simulink model "newsimul"  (R2023a)
settings: Solver=FixedStepAuto  StartTime=0.0  StopTime=51e-6 - 1/2e9  RelTol=1e-3
values from neighbouring files (symbols this model uses):
  yr_c = yr_c(t,:)    [matlab_channel.m]
undefined symbols (not defined in the file or in its folder): Add, Shift
libraries: hdlsllib x3, dsphdlfiltering2 x1, dsphdlmathfun2 x1
settings Model: Creator=Windows User  LastModifiedBy=Windows User
settings OptimizationCC: BlockReduction=off  ConditionallyExecuteInputs=off  DefaultParameterBehavior=Inlined
settings DebuggingCC: AlgebraicLoopMsg=error  SingleTaskRateTransMsg=error
settings HardwareCC: ProdBitPerPointer=32  ProdBitPerSizeT=32  ProdBitPerPtrDiffT=32  ProdLargestAtomicFloat=None  ProdIntDivRoundTo=Undefined  ProdEndianess=Unspecified  ProdWordSize=32  ProdHWDeviceType=ASIC/FPGA->ASIC/FPGA  TargetBitPerPointer=64  TargetBitPerSizeT=64  TargetBitPerPtrDiffT=64  TargetLongLongMode=on  TargetIntDivRoundTo=Zero  TargetEndianess=LittleEndian  TargetWordSize=64  TargetHWDeviceType=Custom Processor->MATLAB Host Computer  ProdEqTarget=off

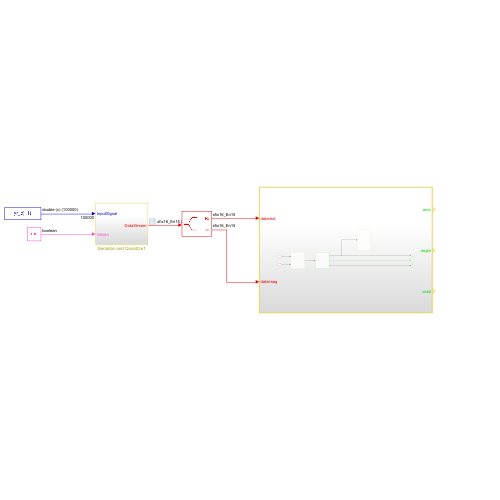
[thumbnail: Simulink's stored preview of the top-level diagram]
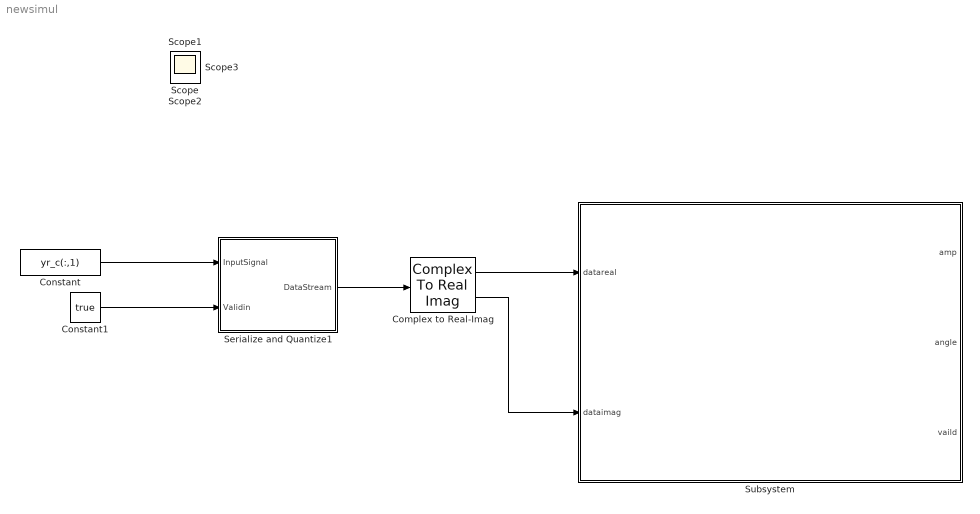
== system newsimul ==
  Complex to Real-Imag : ComplexToRealImag
  Constant : Constant  Value=yr_c(:,1)  SampleTime=50e-6
  Constant1 : Constant  Value=true  OutDataTypeStr=boolean
  Serialize and Quantize1 : Subsystem
  Subsystem : Subsystem  TreatAsAtomicUnit=on
  Scope{,1..3} (4 alike) : Scope
  wires:
  Constant1/1 -> Serialize and Quantize1/2(Validin)
  Serialize and Quantize1/1(DataStream) -> Complex to Real-Imag/1
  Complex to Real-Imag/1 -> Subsystem/1(datareal)
  Complex to Real-Imag/2 -> Subsystem/2(dataimag)
  Constant/1 -> Serialize and Quantize1/1(InputSignal)

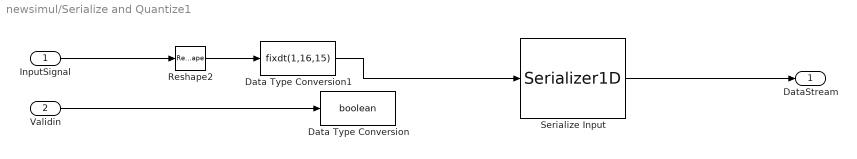
== system newsimul/Serialize and Quantize1 ==
  InputSignal : Inport
  Validin : Inport  Port=2
  Data Type Conversion : DataTypeConversion  OutDataTypeStr=boolean  SaturateOnIntegerOverflow=off  RndMeth=Floor
  Data Type Conversion1 : DataTypeConversion  OutDataTypeStr=fixdt(1,16,15)  RndMeth=Floor
  Reshape2 : Reshape  OutputDimensionality=Column vector (2-D)
  Serialize Input : hdlsllib/HDL Operations/Serializer1D  Ratio=100000  IdleCycles=0  validIn=off  startOut=off  validOut=off  inputDataDimensions=-1  inputSampleTime=-1  inputSignalType=auto
  DataStream : Outport
  wires:
  InputSignal/1 -> Reshape2/1
  Validin/1 -> Data Type Conversion/1
  Serialize Input/1 -> DataStream/1
  Reshape2/1 -> Data Type Conversion1/1
  Data Type Conversion1/1 -> Serialize Input/1

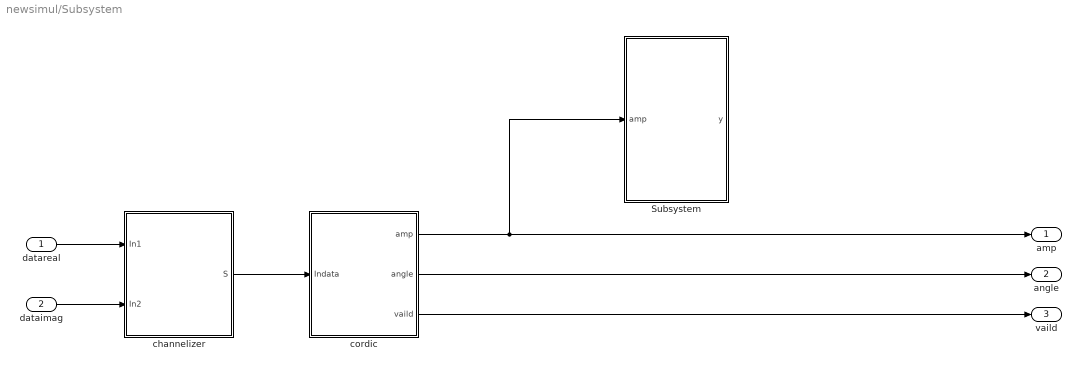
== system newsimul/Subsystem ==
  datareal : Inport
  dataimag : Inport  Port=2
  Subsystem : Subsystem
  channelizer : Subsystem
  cordic : Subsystem
  amp : Outport
  angle : Outport  Port=2
  vaild : Outport  Port=3
  wires:
  datareal/1 -> channelizer/1(In1)
  dataimag/1 -> channelizer/2(In2)
  channelizer/1(S) -> cordic/1(Indata)
  cordic/2(angle) -> angle/1
  cordic/3(vaild) -> vaild/1
  cordic/1(amp) -> amp/1, Subsystem/1(amp)

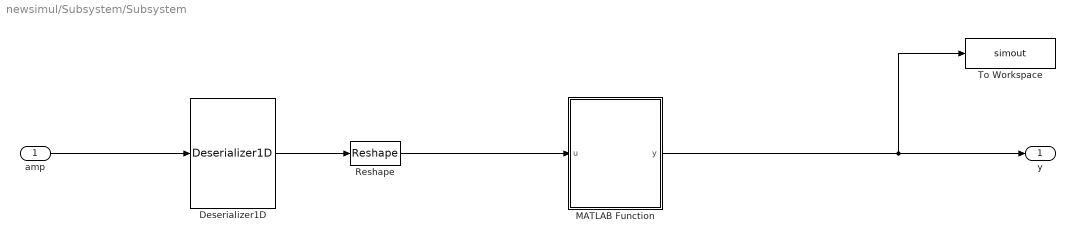
== system newsimul/Subsystem/Subsystem ==
  amp : Inport
  Deserializer1D : hdlsllib/HDL Operations/Deserializer1D  Ratio=100000/32  IdleCycles=0  InitialCondition=0  startIn=off  validIn=off  validOut=off  inputDataDimensions=-1  inputSampleTime=-1  inputSignalType=auto
  MATLAB Function : MATLAB Function  TreatAsAtomicUnit=on
  Reshape : Reshape  OutputDimensionality=Customize  OutputDimensions=[32,100000/32]
  To Workspace : ToWorkspace  VariableName=simout  SampleTime=-1
  y : Outport
  wires:
  amp/1 -> Deserializer1D/1
  Deserializer1D/1 -> Reshape/1
  MATLAB Function/1(y) -> To Workspace/1, y/1
  Reshape/1 -> MATLAB Function/1(u)

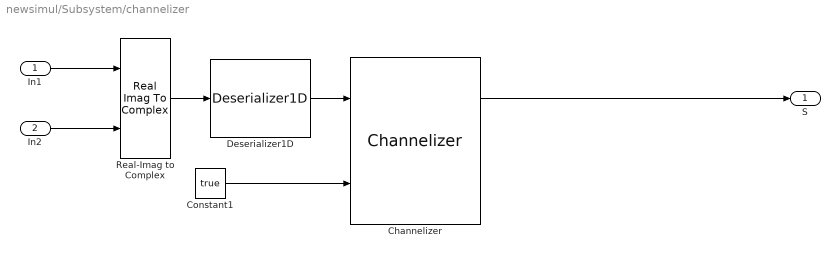
== system newsimul/Subsystem/channelizer ==
  In1 : Inport
  In2 : Inport  Port=2
  Channelizer : dsphdlfiltering2/Channelizer  FilterCoefficients=LowpassCoefficients  FilterStructure=Direct form transposed  NumFrequencyBands=FFTLength  ComplexMultiplication=Use 4 multipliers and 2 adders  Normalize=on  OutputSize=Same as input size  SimulateUsing=Code generation  roundingMode=Floor  overflowMode=off  CoefficientsDataTypeStr=Inherit: Same word length as input  FilterOutputDataTypeStr=fixdt(1,16,15)  ResetInputPort=off  StartOutputPort=off  EndOutputPort=off
  Constant1 : Constant  Value=true  OutDataTypeStr=boolean
  Deserializer1D : hdlsllib/HDL Operations/Deserializer1D  Ratio=FFTLength  IdleCycles=0  InitialCondition=0  startIn=off  validIn=off  validOut=off  inputDataDimensions=-1  inputSampleTime=-1  inputSignalType=auto
  Real-Imag to Complex : RealImagToComplex
  S : Outport
  wires:
  In2/1 -> Real-Imag to Complex/2
  Deserializer1D/1 -> Channelizer/1
  Real-Imag to Complex/1 -> Deserializer1D/1
  In1/1 -> Real-Imag to Complex/1
  Constant1/1 -> Channelizer/2
  Channelizer/1 -> S/1

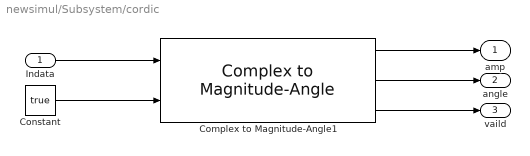
== system newsimul/Subsystem/cordic ==
  Indata : Inport
  Complex to Magnitude-Angle1 : dsphdlmathfun2/Complex to Magnitude-Angle  NumIterationsSource=Property  NumIterations=15  OutputFormat=Magnitude and angle  AngleFormat=Radians  ScaleOutput=on  ScalingMethod=Shift-Add  SimulateUsing=Code generation
  Constant : Constant  Value=true  OutDataTypeStr=boolean  SampleTime=-1
  amp : Outport
  angle : Outport  Port=2
  vaild : Outport  Port=3
  wires:
  Indata/1 -> Complex to Magnitude-Angle1/1
  Complex to Magnitude-Angle1/1 -> amp/1
  Constant/1 -> Complex to Magnitude-Angle1/2
  Complex to Magnitude-Angle1/2 -> angle/1
  Complex to Magnitude-Angle1/3 -> vaild/1

== matlab function newsimul/Subsystem/Subsystem/MATLAB Function ==
  data: u input; y output
function y = fcn(u)
average_data = sum(u)/32;
data_cha = u - average_data;

y = zeros(32,5);


for i = 1:32
    up_times = 0;%记录上升次数
    down_times = 0;%记录下降次数
    up = 0;%上升标志
    down = 0;%下降标志
    time = 0;%计时
    for j = 1:100000/32
        if data_cha(i,j) > 0
            up_times = up_times + 1;
            down_times = 0;
        else
            up_times = 0;
            down_times = down_times + 1;
        end
        
        if up == 0 && up_times >20
            up = time;
            down = 100000/32;
        end

        if down == 100000/32 && down_times >20
            down = time;
        end

        time = time + 1;
    end

    if up == 0
        y(i,1) = i;%通道号
        y(i,2) = 0;%无脉冲
        y(i,3) = 0;%脉宽为0；
        y(i,4) = up;
        y(i,5) = down;
    else
        y(i,1) = i;
        y(i,2) = 1;
        y(i,3) = 16*(down-up)/1e6;
        y(i,4) = up;
        y(i,5) = down;
    end

end







%y = data_cha;
